simulink model "SILTopModel"  (R2022b)
settings: Solver=FixedStepDiscrete  StartTime=0.0  StopTime=10.0  FixedStep=T  RelTol=1e-3  EnableMultiTasking=on
PostLoadFcn:
  | rtwdemo_overrides={'CodeProfilingInstrumentation','CodeProfilingSaveOptions','CodeExecutionProfiling','LaunchReport','PassReuseOutputArgsAs', 'GenerateCodeMetricsReport','ProdHWDeviceType','PortableWordSizes','ProdIntDivRoundTo'};
  | rtwconfiguredemo(gcs,'ERT',rtwdemo_overrides{:});
  | clear rtwdemo_overrides
  | 
  | % Code coverage settings
  | ldraPath = '';
  | bullseyePath = '';
  | try
  |     ldraPath = coder.coverage.LDRA.getPath;
  |     bullseyePath = coder.coverage.BullseyeCoverage.getPath;
  | catch e
  |     % It is possible that the code coverage tool path is no longer valid
  |     if ~strcmp(e.identifier, 'CoderCoverage:AllTools:toolPathGetInvalid')
  |         rethrow(e)
  |     end
  |     % Clear exception variable
  |     clear e
  | end
  | 
  | coverageSettings = get_param(gcs,'CodeCoverageSettings');
  | coverageSettings.TopModelCoverage='on';
  | coverageSettings.CoverageTool='None';
  | if ~isempty(ldraPath)
  |     coverageSettings.CoverageTool='LDRAcover or LDRA tool suite';
  |     %Disable sample main generation when Coverage Enabled
  |     set_param(gcs,'GenerateSampleERTMain','off');
  | elseif ~isempty(bullseyePath)
  |     coverageSettings.CoverageTool='BullseyeCoverage';
  |     %Disable sample main generation when Coverage Enabled
  |     set_param(gcs,'GenerateSampleERTMain','off');
  | else
  |     coverageSettings.CoverageTool='None';
  | end
  | set_param(gcs, 'CodeCoverageSettings', coverageSettings);
  | 
  | % Default to SIL simulation mode
  | set_param(gcs,'SimulationMode','software-in-the-loop')
  | 
  | % Ensure the Simulation Data Inspector is opened automatically
  | set_param(gcs, 'InspectSignalLogs', 'on');
  | 
  | % Sample time
  | T=0.1;
  | [ticks_to_count, reset, counter_mode, count_enable, ...
  |         counter_mode_values_run1, counter_mode_values_run2, ...
  |         count_enable_values_run1, count_enable_values_run2] = ...
  |         SILTopModelData(T);
  | 
  | % Parameters
  | countUpper = uint8(40);
  | countLower = uint8(20);
  | counter_mode_select = 0;
Description:
  | A top model for software-in-the-loop (SIL) or processor-in-the-loop (PIL) examples.
settings Model: FPTRunName=Active  SimulationMode=software-in-the-loop (sil)  Creator=The MathWorks, Inc.  LastModifiedBy=The MathWorks, Inc.
settings SolverCC: AlgebraicLoopSolver=TrustRegion  MaxZcPerStep=1
settings DataIOCC: ExternalInput=ticks_to_count, reset, counter_mode, count_enable  LoadExternalInput=on  SaveFormat=StructureWithTime  SaveOutput=off  DSMLogging=off  InspectSignalLogs=on  SaveTime=off  SignalLoggingName=logsOut
settings OptimizationCC: DefaultParameterBehavior=Inlined  UseDivisionForNetSlopeComputation=on  InlineInvariantSignals=on  EnhancedBackFolding=on  BooleansAsBitfields=on  PassReuseOutputArgsAs=Individual arguments  ExpressionDepthLimit=2147483647  StateBitsets=on  DataBitsets=on  ZeroExternalMemoryAtStartup=off  ZeroInternalMemoryAtStartup=off  NoFixptDivByZeroProtection=on  EfficientFloat2IntCast=on  SimCompilerOptimization=on  OptimizeBlockOrder=speed  DifferentSizesBufferReuse=on  EfficientTunableParamExpr=on
settings DebuggingCC: ReadBeforeWriteMsg=DisableAll  WriteAfterWriteMsg=DisableAll  WriteAfterReadMsg=DisableAll  CheckExecutionContextPreStartOutputMsg=on  ParameterTunabilityLossMsg=error  FcnCallInpInsideContextMsg=warning  UnconnectedInputMsg=warning  UnconnectedOutputMsg=warning  UnconnectedLineMsg=warning  UniqueDataStoreMsg=error  AllowSymbolicDim=off  ModelReferenceSymbolNameMessage=none  StateNameClashWarn=warning  StrictBusMsg=ErrorOnBusTreatedAsVector  SFUnexpectedBacktrackingDiag=warning  SFNoUnconditionalDefaultTransitionDiag=warning  SFExecutionAtInitializationDiag=none  SFMachineParentedDataDiag=warning  ArithmeticOperatorsInVariantConditions=warning
settings HardwareCC: ProdBitPerPointer=32  ProdBitPerSizeT=32  ProdBitPerPtrDiffT=32  ProdLargestAtomicInteger=Long  ProdLargestAtomicFloat=Double  ProdWordSize=32  ProdHWDeviceType=ARM Compatible->ARM Cortex  TargetHWDeviceType=Generic->32-bit Embedded Processor
settings ModelReferenceCC: EnableRefExpFcnMdlSchedulingChecks=on  CheckModelReferenceTargetMessage=none  ModelReferencePassRootInputsByReference=off  PropagateSignalLabelsOutOfModel=off
settings SFSimCC: SimUseLocalCustomCode=off  MATLABDynamicMemAlloc=off  CustomCodeUndefinedFunction=UseInterfaceOnly
settings RTWCC: Description=Embedded Coder  SystemTargetFile=ert.tlc  TLCOptions=-p0 -aWarnNonSaturatedBlocks=0  TemplateMakefile=ert_default_tmf  GenerateReport=on  RTWVerbose=off  RTWUseLocalCustomCode=off  IncludeHyperlinkInReport=on  PortableWordSizes=on  CodeExecutionProfiling=on  CodeProfilingSaveOptions=AllData  GenerateTraceInfo=on  GenerateTraceReport=on  GenerateTraceReportSl=on  GenerateTraceReportSf=on  GenerateTraceReportEml=on  DLArmComputeVersion=19.05
settings CodeAppCC: ForceParamTrailComments=on  IgnoreCustomStorageClasses=off  OperatorAnnotations=on  SimulinkDataObjDesc=on  SFDataObjDesc=on  CustomSymbolStrGlobalVar=rt$N$M  CustomSymbolStrType=$N$M  CustomSymbolStrFcn=$N$M$F  CustomSymbolStrModelFcn=$N  CustomSymbolStrMacro=$N$M  InsertBlockDesc=on  InternalIdentifier=Classic
settings ERTTargetCC: UtilityFuncGeneration=Shared location  GenerateSampleERTMain=on  IncludeMdlTerminateFcn=off  CombineSignalStateStructs=on  SupportNonFinite=off  SupportComplex=off  InlinedParameterPlacement=NonHierarchical  ERTCustomFileTemplate=example_file_process.tlc  ERTFilePackagingFormat=CompactWithDataFile
settings ConfigComp: CovEnable=on  CovScope=ReferencedModels  RecordCoverage=on  CovCompData=covCumulativeData  CovMetricSettings=dcmrswe  CovHTMLOptions=-aTS=1 -bRG=1 -bTC=1 -hTR=0 -nFC=0 -scm=1 -bcm=1 -xEv=0  CovSaveCumulativeToWorkspaceVar=on  CovSaveSingleToWorkspaceVar=on  CovCumulativeReport=on  CovExternalEMLEnable=off

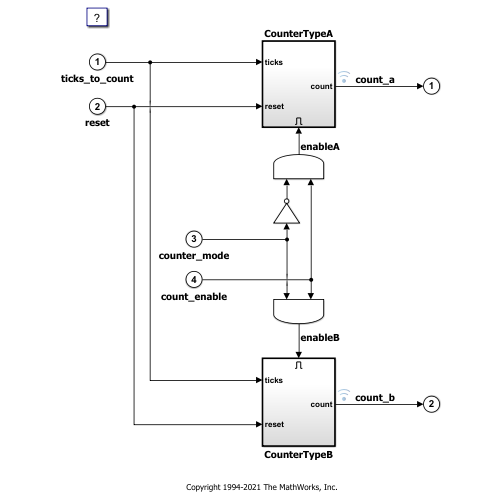
[thumbnail: Simulink's stored preview of the top-level diagram]
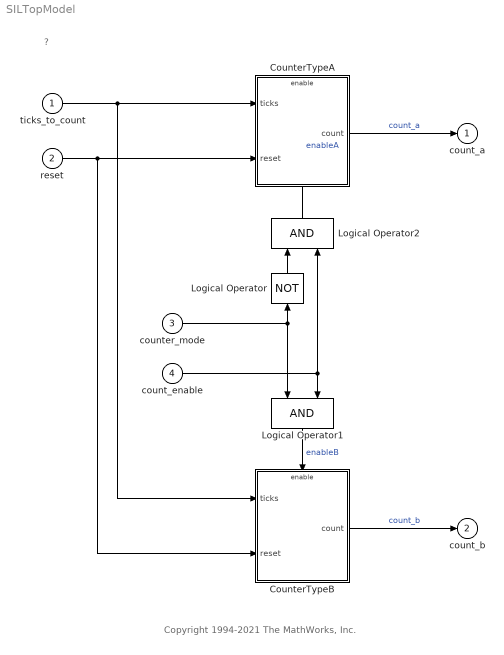
== system SILTopModel ==
  note: Copyright 1994-2021 The MathWorks, Inc.
  note: ?
  ticks_to_count : Inport  OutDataTypeStr=boolean  PortDimensions=1  SampleTime=T
  reset : Inport  Port=2  OutDataTypeStr=boolean  PortDimensions=1  SampleTime=T
  counter_mode : Inport  Port=3  OutDataTypeStr=boolean  PortDimensions=1  SampleTime=T
  count_enable : Inport  Port=4  OutDataTypeStr=boolean  PortDimensions=1  SampleTime=T
  CounterTypeA : Subsystem
      settings: RTWSystemCode=Nonreusable function  RTWFcnNameOpts=Use subsystem name
  CounterTypeB : Subsystem
      settings: RTWSystemCode=Nonreusable function  RTWFcnNameOpts=Use subsystem name
  Logical Operator : Logic  Operator=NOT  IconShape=distinctive  AllPortsSameDT=off  OutDataTypeStr=boolean
  Logical Operator1 : Logic  IconShape=distinctive  AllPortsSameDT=off  OutDataTypeStr=boolean
  Logical Operator2 : Logic  IconShape=distinctive  AllPortsSameDT=off  OutDataTypeStr=boolean
  count_a : Outport  VectorParamsAs1DForOutWhenUnconnected=off
  count_b : Outport  Port=2  VectorParamsAs1DForOutWhenUnconnected=off
  wires:
  ticks_to_count/1 -> CounterTypeA/1(ticks), CounterTypeB/1(ticks)
  reset/1 -> CounterTypeA/2(reset), CounterTypeB/2(reset)
  CounterTypeA/1(count) -> count_a/1  "count_a"
  CounterTypeB/1(count) -> count_b/1  "count_b"
  Logical Operator1/1 -> CounterTypeB/Enable  "enableB"
  Logical Operator2/1 -> CounterTypeA/Enable  "enableA"
  Logical Operator/1 -> Logical Operator2/1
  counter_mode/1 -> Logical Operator1/1, Logical Operator/1
  count_enable/1 -> Logical Operator1/2, Logical Operator2/2

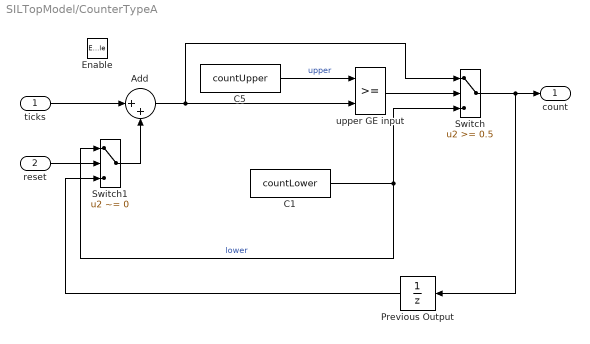
== system SILTopModel/CounterTypeA ==
  ticks : Inport
  reset : Inport  Port=2
  Enable : EnablePort
  Add : Sum  Inputs=|++  OutDataTypeStr=uint8
  C1 : Constant  Value=countLower  OutDataTypeStr=uint8
  C5 : Constant  Value=countUpper  OutDataTypeStr=uint8
  Previous Output : UnitDelay  InitialCondition=25  SampleTime=T  HasFrameUpgradeWarning=on
  Switch : Switch  Threshold=0.5  SaturateOnIntegerOverflow=off
  Switch1 : Switch  Criteria=u2 ~= 0  Threshold=0.5  SaturateOnIntegerOverflow=off
  upper GE input : RelationalOperator  Priority=0  OutDataTypeStr=boolean
      settings: AttributesFormatString=\n
  count : Outport  InitialOutput=25  VectorParamsAs1DForOutWhenUnconnected=off
  wires:
  Switch/1 -> Previous Output/1, count/1
  upper GE input/1 -> Switch/2
  C5/1 -> upper GE input/1  "upper"
  Add/1 -> upper GE input/2, Switch/1
  C1/1 -> Switch/3, Switch1/1  "lower"
  Previous Output/1 -> Switch1/3
  Switch1/1 -> Add/2
  ticks/1 -> Add/1
  reset/1 -> Switch1/2

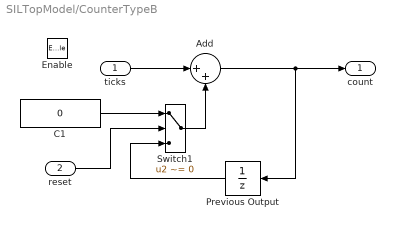
== system SILTopModel/CounterTypeB ==
  ticks : Inport
  reset : Inport  Port=2
  Enable : EnablePort
  Add : Sum  Inputs=|++  OutDataTypeStr=uint8
  C1 : Constant  Value=0  OutDataTypeStr=uint8
  Previous Output : UnitDelay  InitialCondition=15  SampleTime=T  HasFrameUpgradeWarning=on
  Switch1 : Switch  Criteria=u2 ~= 0  Threshold=0.5  SaturateOnIntegerOverflow=off
  count : Outport  InitialOutput=15  VectorParamsAs1DForOutWhenUnconnected=off
  wires:
  ticks/1 -> Add/1
  reset/1 -> Switch1/2
  Switch1/1 -> Add/2
  Previous Output/1 -> Switch1/3
  Add/1 -> count/1, Previous Output/1
  C1/1 -> Switch1/1
